simulink model "symulacja_ryb"  (R2023b)
settings: Solver=VariableStepAuto  StartTime=0.0  StopTime=600  RelTol=1e-3
settings Model: Creator=z1186362  LastModifiedBy=msztu223

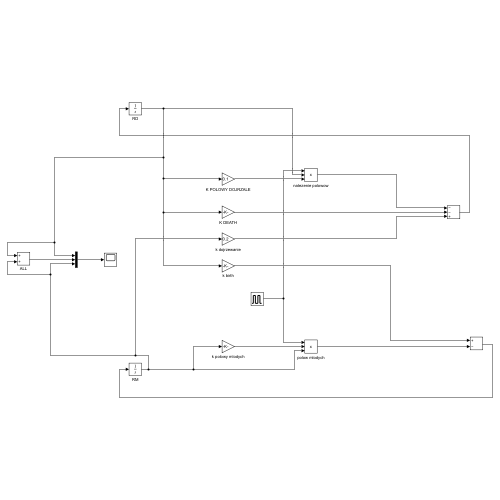
[thumbnail: Simulink's stored preview of the top-level diagram]
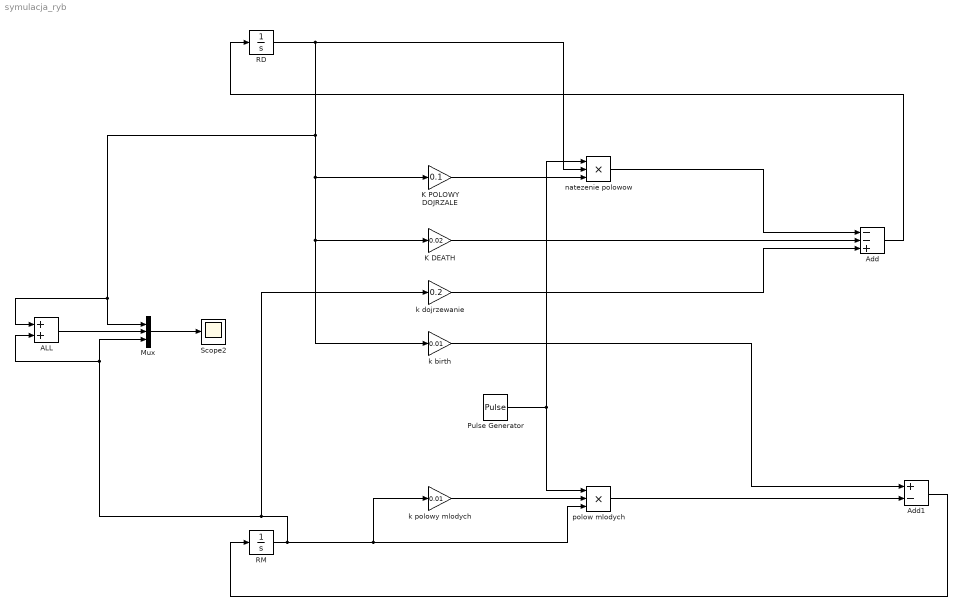
== system symulacja_ryb ==
  ALL : Sum
  Add : Sum  Inputs=--+
  Add1 : Sum  Inputs=+-
  K DEATH : Gain  Gain=0.02
  K POLOWY DOJRZALE : Gain  Gain=0.1
  Mux : Mux  Inputs=3
  Pulse Generator : DiscretePulseGenerator  PulseType=Time based  Amplitude=0.1  Period=12  PulseWidth=10
  RD : Integrator  InitialCondition=100
  RM : Integrator  InitialCondition=40
  Scope2 : Scope
  k birth : Gain  Gain=0.01
  k dojrzewanie : Gain  Gain=0.2
  k polowy mlodych : Gain  Gain=0.01
  natezenie polowow : Product  Inputs=3
  polow mlodych : Product  Inputs=3
  wires:
  RD/1 -> Mux/1, ALL/1, k birth/1, K DEATH/1, K POLOWY DOJRZALE/1, natezenie polowow/2
  K POLOWY DOJRZALE/1 -> natezenie polowow/3
  Add/1 -> RD/1
  k birth/1 -> Add1/1
  RM/1 -> Mux/3, ALL/2, k dojrzewanie/1, k polowy mlodych/1, polow mlodych/3
  polow mlodych/1 -> Add1/2
  Add1/1 -> RM/1
  k dojrzewanie/1 -> Add/3
  K DEATH/1 -> Add/2
  natezenie polowow/1 -> Add/1
  Pulse Generator/1 -> polow mlodych/1, natezenie polowow/1
  Mux/1 -> Scope2/1
  ALL/1 -> Mux/2
  k polowy mlodych/1 -> polow mlodych/2
